simulink subsystem "ControlledCurrentSource"  (R2025a)
settings: Solver=VariableStepAuto  StartTime=0.0  StopTime=10.0  RelTol=1e-3
model mask{I_max=0, I_min=0}
  mask prompts: I_max "Current Upper limit (A):"; I_min "Current Lower limit (A):"
libraries: fl_lib x3, nesl_utility x2
settings Model: Creator=Polarstern  LastModifiedBy=CelestialAurora

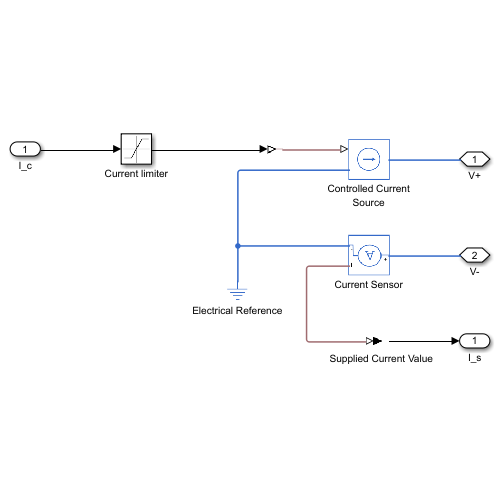
[thumbnail: Simulink's stored preview of the top-level diagram]
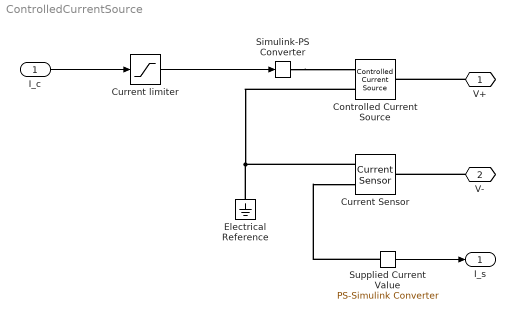
== system ControlledCurrentSource ==
  I_c : Inport
  Controlled Current Source : fl_lib/Electrical/Electrical Sources/Controlled Current Source
  Current Sensor : fl_lib/Electrical/Electrical Sensors/Current Sensor
  Current limiter : Saturate  UpperLimit=I_max  LowerLimit=I_min
  Electrical Reference : fl_lib/Electrical/Electrical Elements/Electrical Reference
  Simulink-PS Converter : nesl_utility/Simulink-PS Converter  PhysicalDomain=network_engine_domain  SubClassName=ps_input  LeftPortType=input  RightPortType=output  PseudoPeriodic=off  Frequencies=[]  NoiseDistribution=none  NoiseParameters=[]  Unit=1  AffineConversion=off  FilteringAndDerivatives=zero  SimscapeFilterOrder=1  InputFilterTimeConstant=0.001  UdotUserProvided=0
  Supplied Current Value : nesl_utility/PS-Simulink Converter  PhysicalDomain=network_engine_domain  SubClassName=ps_output  LeftPortType=input  RightPortType=output  PseudoPeriodic=off  Frequencies=[]  VectorFormat=inherit  Unit=inherit  AffineConversion=off
  V+ : PMIOPort  Side=Right
  V- : PMIOPort  Port=2  Side=Right
  I_s : Outport
  wires:
  I_c/1 -> Current limiter/1
  Current limiter/1 -> Simulink-PS Converter/1
  Supplied Current Value/1 -> I_s/1
  connections:
  Controlled Current Source/RConn2 -- Electrical Reference/LConn1 -- Current Sensor/RConn2
  V+/RConn1 -- Controlled Current Source/LConn1
  Simulink-PS Converter/RConn1 -- Controlled Current Source/RConn1
  V-/RConn1 -- Current Sensor/LConn1
  Supplied Current Value/LConn1 -- Current Sensor/RConn1
